simulink model "ElMejor"  (R2017a)
settings: Solver=VariableStepAuto  StartTime=0.0  StopTime=0.8  RelTol=1e-3
values from neighbouring files (symbols this model uses):
  C = 33e-6    (= 3.3e-05)    [Practica_1.m]
  Kd = ((1 + Kp)/(2*P*Wn)) - (R*C)    [Practica_1.m]
  Ki = ((Wn)^2)*(R*C + Kd)    [Practica_1.m]
  Kp = 0.74    [Practica_1.m]
  Kw = 2    [Practica_1.m]
  R = 1e3    (= 1000)    [Practica_1.m]
settings Model: Creator=LuisCarlos  LastModifiedBy=LuisCarlos

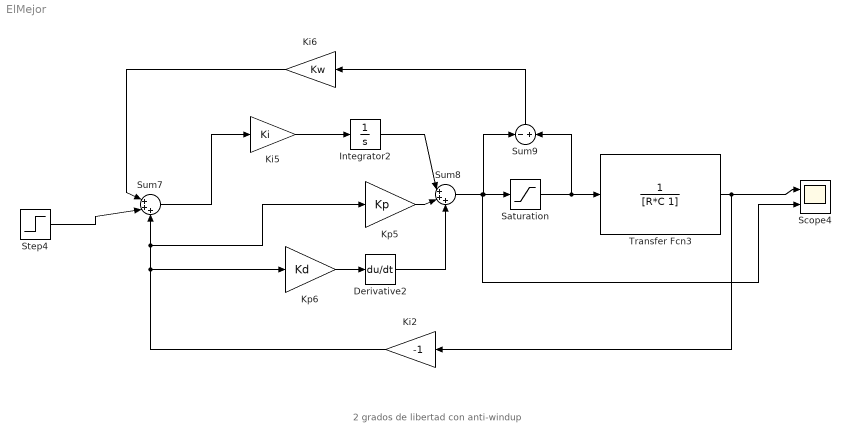
== system ElMejor ==
  note: 2 grados de libertad con anti-windup
  Derivative2 : Derivative
  Integrator2 : Integrator
  Ki2 : Gain  Gain=-1
  Ki5 : Gain  Gain=Ki
  Ki6 : Gain  Gain=Kw
  Kp5 : Gain  Gain=Kp
  Kp6 : Gain  Gain=Kd
  Saturation : Saturate  UpperLimit=5  LowerLimit=0
  Scope4 : Scope  NumInputPorts=2
  Step4 : Step  Time=0  After=3.3  SampleTime=0
  Sum7 : Sum  Inputs=|+++
  Sum8 : Sum  Inputs=|+++
  Sum9 : Sum  Inputs=-+
  Transfer Fcn3 : TransferFcn  Denominator=[R*C 1]
  wires:
  Ki6/1 -> Sum7/1
  Sum9/1 -> Ki6/1
  Integrator2/1 -> Sum8/1
  Kp5/1 -> Sum8/2
  Ki5/1 -> Integrator2/1
  Kp6/1 -> Derivative2/1
  Derivative2/1 -> Sum8/3
  Ki2/1 -> Sum7/3, Kp5/1, Kp6/1
  Transfer Fcn3/1 -> Ki2/1, Scope4/1
  Sum7/1 -> Ki5/1
  Sum8/1 -> Scope4/2, Sum9/1, Saturation/1
  Step4/1 -> Sum7/2
  Saturation/1 -> Sum9/2, Transfer Fcn3/1
